simulink model "NonLinearVehicleiLQR"  (R2020b)
settings: Solver=FixedStepDiscrete  StartTime=0.0  StopTime=20  FixedStep=0.001  MaxStep=0.01  RelTol=1e-3
undefined symbols (not defined in the file): b, DiscIntNeverNeededParam, Q, Qf, R, r
libraries: simulink x1
settings Model: Creator=iris  LastModifiedBy=iris

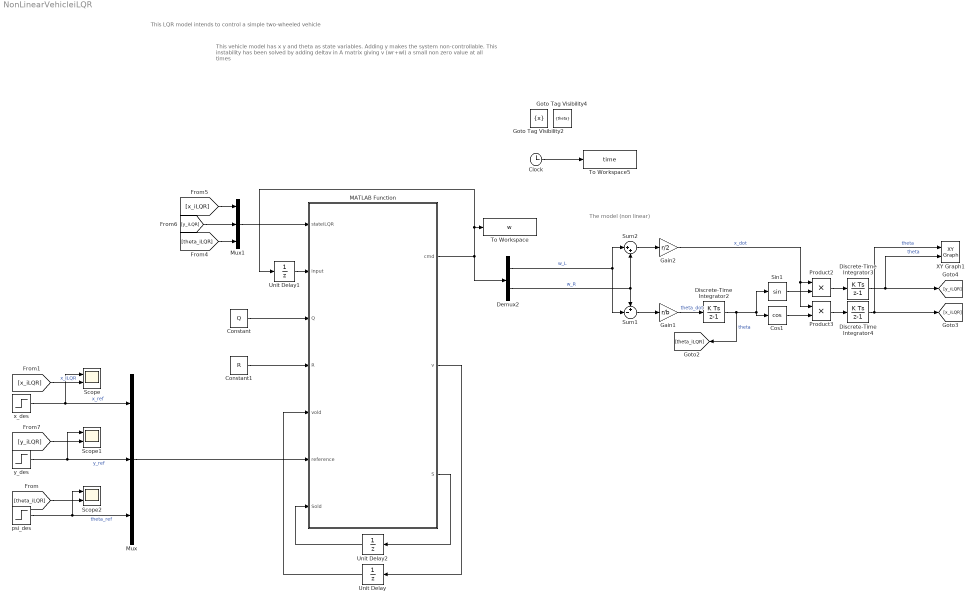
== system NonLinearVehicleiLQR ==
  note: The model (non linear)
  note: This vehicle model has x y and theta as state variables. Adding y makes the system non-controllable. This instability has been solved by adding deltav in A matrix giving v (wr+wl) a small non zero value at all times
  note: This LQR model intends to control a simple two-wheeled vehicle
  Clock : Clock
  Constant : Constant  Value=Q
  Constant1 : Constant  Value=R
  Cos1 : Trigonometry  Operator=cos
  Demux2 : Demux  Outputs=2
  Discrete-Time Integrator2 : DiscreteIntegrator  SampleTime=-1  ICPrevOutput=DiscIntNeverNeededParam  ICPrevScaledInput=DiscIntNeverNeededParam
  Discrete-Time Integrator3 : DiscreteIntegrator  SampleTime=-1  ICPrevOutput=DiscIntNeverNeededParam  ICPrevScaledInput=DiscIntNeverNeededParam
  Discrete-Time Integrator4 : DiscreteIntegrator  SampleTime=-1  ICPrevOutput=DiscIntNeverNeededParam  ICPrevScaledInput=DiscIntNeverNeededParam
  Gain1 : Gain  Gain=r/b
  Gain2 : Gain  Gain=r/2
  Goto Tag Visibility2 : GotoTagVisibility  GotoTag=x
  Goto Tag Visibility4 : GotoTagVisibility  GotoTag=theta
  MATLAB Function : MATLAB Function  TreatAsAtomicUnit=on
  Mux : Mux  Inputs=3
  Mux1 : Mux  Inputs=3
  Product2 : Product
  Product3 : Product
  Scope : Scope  NumInputPorts=2
  Scope1 : Scope  NumInputPorts=2
  Scope2 : Scope  NumInputPorts=2
  Sin1 : Trigonometry
  Sum1 : Sum  Inputs=+-|
  Sum2 : Sum  Inputs=|++
  To Workspace : ToWorkspace  VariableName=w  SampleTime=-1
  To Workspace5 : ToWorkspace  VariableName=time  SampleTime=-1
  Unit Delay : UnitDelay  InitialCondition=zeros(3,1)  SampleTime=-1  HasFrameUpgradeWarning=on
  Unit Delay1 : UnitDelay  InitialCondition=[0, 0]  SampleTime=-1  HasFrameUpgradeWarning=on
  Unit Delay2 : UnitDelay  InitialCondition=Qf  SampleTime=-1  HasFrameUpgradeWarning=on
  XY Graph1 : simulink/Sinks/XY Graph  xmin=-2  xmax=2  ymin=-2  ymax=2  st=-1
  psi_des : Step  Time=0  After=0  SampleTime=0
  x_des : Step  Time=3  SampleTime=0
  y_des : Step  Time=0  SampleTime=0
  wires:
  MATLAB Function/3(S) -> Unit Delay2/1
  Unit Delay2/1 -> MATLAB Function/7(Sold)
  MATLAB Function/2(v) -> Unit Delay/1
  Unit Delay/1 -> MATLAB Function/5(vold)
  MATLAB Function/1(cmd) -> Unit Delay1/1, To Workspace/1, Demux2/1
  Constant/1 -> MATLAB Function/3(Q)
  Constant1/1 -> MATLAB Function/4(R)
  Mux/1 -> MATLAB Function/6(reference)
  x_des/1 -> Scope/1, Mux/1  "x_ref"
  psi_des/1 -> Scope2/1, Mux/3  "theta_ref"
  Clock/1 -> To Workspace5/1
  Unit Delay1/1 -> MATLAB Function/2(input)
  [x_iLQR] -> Scope/2  "x_iLQR"
  [theta_iLQR] -> Scope2/2
  Gain1/1 -> Discrete-Time Integrator2/1  "theta_dot"
  Sum1/1 -> Gain1/1
  Demux2/1 -> Sum2/1, Sum1/2  "w_L"
  Demux2/2 -> Sum2/2, Sum1/1  "w_R"
  Sum2/1 -> Gain2/1
  Mux1/1 -> MATLAB Function/1(stateiLQR)
  [x_iLQR] -> Mux1/1
  [theta_iLQR] -> Mux1/3
  Gain2/1 -> Product3/1, Product2/1  "x_dot"
  Product3/1 -> Discrete-Time Integrator4/1
  Sin1/1 -> Product2/2
  Discrete-Time Integrator2/1 -> Sin1/1, Cos1/1, [theta_iLQR]  "theta"
  Cos1/1 -> Product3/2
  Product2/1 -> Discrete-Time Integrator3/1
  [y_iLQR] -> Mux1/2
  Discrete-Time Integrator3/1 -> XY Graph1/2, [y_iLQR]  "theta"
  Discrete-Time Integrator4/1 -> XY Graph1/1, [x_iLQR]  "theta"
  [y_iLQR] -> Scope1/2
  y_des/1 -> Scope1/1, Mux/2  "y_ref"

== matlab function NonLinearVehicleiLQR/MATLAB Function ==
  data: stateiLQR input; cmd output; input input; Q input; R input; vold input; reference input; Sold input; v output; S output
function [cmd, v, S]= fcn(stateiLQR, input , Q, R, vold, reference, Sold)

r = 0.02;
b = 0.185;
dt = 0.001;

% toll = 3*10^-5;

% A = [1 0 dt*-sin(psi)*r/2*(wR+wL);...
%      0 1 dt*cos(psi)*r/2*(wR+wL);...
%      0 0 1];
% B = dt*[cos(psi)*r/2 cos(psi)*r/2;...
%      sin(psi)*r/2 sin(psi)*r/2;...
%      -r/b r/b];
% A = eye(3);
% B = dt*[r/2 r/2;
%      0 0;
%      -r/b r/b];
deltav = 0.00001; % this ensures the system is controllable everytime
% A = [1 0 dt*-sin(psi)*r/2*(wR+wL+deltav);...
%      0 1 dt*cos(psi)*r/2*(wR+wL+deltav);...
%      0 0 1];
% B = dt*[cos(psi)*r/2 cos(psi)*r/2;...
%      sin(psi)*r/2 sin(psi)*r/2;...
%      -r/b r/b];
% A = [1 dt*r/2*(sum(input));
%     0 1];
% B = dt*[r/2 r/2;
%     -r/b r/b];

state = stateiLQR';
psi = stateiLQR(3);
wR = input(2);
wL = input(1);
A = [1 0 dt*-sin(psi)*r/2*(wR+wL+deltav);...
     0 1 dt*cos(psi)*r/2*(wR+wL+deltav);...
     0 0 1];
B = dt*[cos(psi)*r/2 cos(psi)*r/2;...
     sin(psi)*r/2 sin(psi)*r/2;...
     -r/b r/b];
 
K  = (B'*Sold*B+R)\B'*Sold*A;
Kv = (B'*Sold*B+R)\B';
Ku = (B'*Sold*B+R)\R;
S  = A'*Sold*(A-B*K)+Q;
deltax = -reference; % Changed the sign on this one because
% otherwise, the state is mirrored to the reference
v  = (A-B*K)'*vold+Q*deltax-K'*R*input;
deltau = -K*state'-Kv*v-Ku*input;
cmd  = input + deltau;

end
